simulink model "Second_ODE"  (R2019a)
settings: Solver=VariableStepAuto  StartTime=0.0  StopTime=10.0  RelTol=1e-3
undefined symbols (not defined in the file): b, G, k, M
settings Model: Creator=Mahe  LastModifiedBy=Mahe

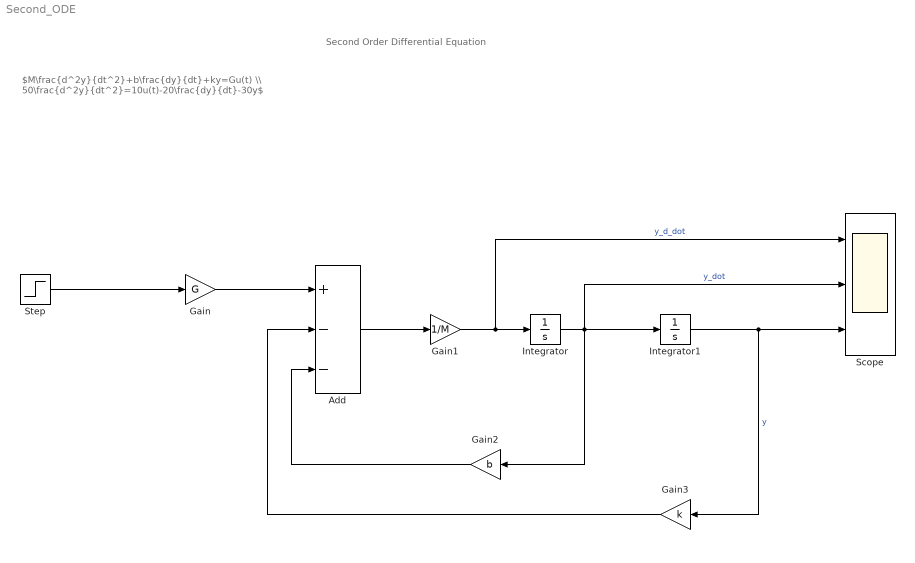
== system Second_ODE ==
  note: Second Order Differential Equation
  note: $M\frac{d^2y}{dt^2}+b\frac{dy}{dt}+ky=Gu(t) \\ 50\frac{d^2y}{dt^2}=10u(t)-20\frac{dy}{dt}-30y$
  Add : Sum  Inputs=+--
  Gain : Gain  Gain=G
  Gain1 : Gain  Gain=1/M
  Gain2 : Gain  Gain=b
  Gain3 : Gain  Gain=k
  Integrator : Integrator
  Integrator1 : Integrator
  Scope : Scope  NumInputPorts=3
  Step : Step  Time=0  SampleTime=0
  wires:
  Gain/1 -> Add/1
  Step/1 -> Gain/1
  Add/1 -> Gain1/1
  Gain1/1 -> Scope/1, Integrator/1  "y_d_dot"
  Integrator/1 -> Gain2/1, Scope/2, Integrator1/1  "y_dot"
  Integrator1/1 -> Gain3/1, Scope/3  "y"
  Gain2/1 -> Add/3
  Gain3/1 -> Add/2
